simulink model "mult_signal"  (R2023a)
settings: Solver=FixedStepAuto  StartTime=0.0  StopTime=50.0  FixedStep=1e-5  RelTol=1e-3
undefined symbols (not defined in the file): LF, sample
libraries: instrumentseriallib x3
settings Model: Creator=Aliso  LastModifiedBy=Aliso

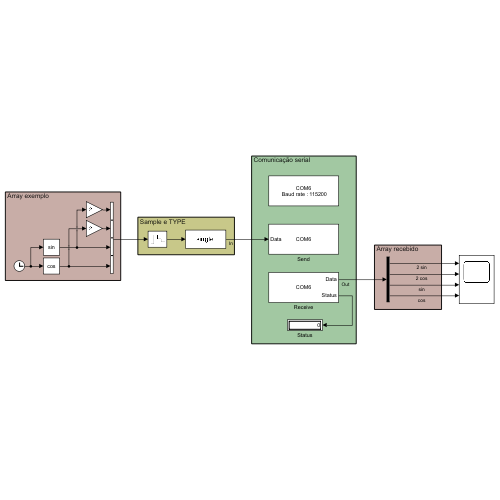
[thumbnail: Simulink's stored preview of the top-level diagram]
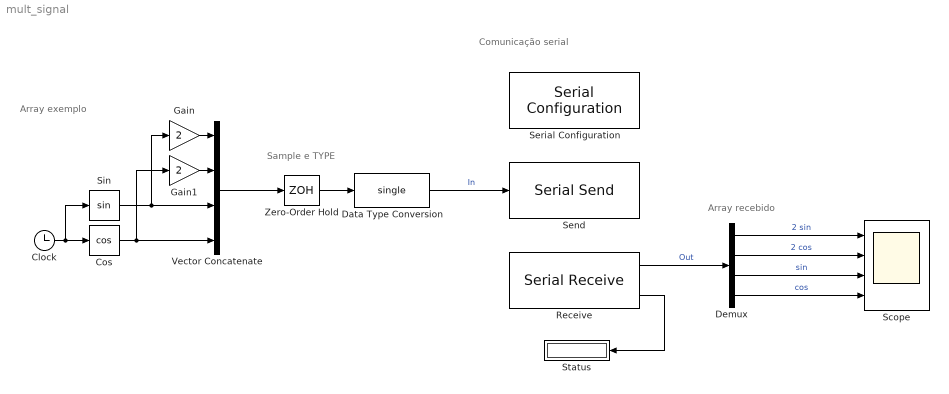
== system mult_signal ==
  note: Comunicação serial
  note: Array recebido
  note: Sample e TYPE
  note: Array exemplo
  Clock : Clock
  Cos : Trigonometry  Operator=cos
  Data Type Conversion : DataTypeConversion  OutDataTypeStr=single  SaturateOnIntegerOverflow=off  RndMeth=Floor  LockScale=on
  Demux : Demux
  Gain : Gain  Gain=2
  Gain1 : Gain  Gain=2
  Receive : instrumentseriallib/Serial Receive  Priority=1  PortSel=COM6  Port=COM6  ComPort=COM6  DataType=single  SaveDataType=uint8  ToggleHeader=on  Header=[65]  ToggleTerminator=on  Terminator=LF ('\n')  CustomTerminator=[]  InputFormat=Column major  ToggleDataSize=on  DataSize=[1 4]  EnableBlockingMode=off  ActionDataUnavailable=Output last received value  ActionWhenDataUnavailable=Output last received value  CustomValue=0  SampleTime=sample/2  SimulateUsing=Interpreted execution  BlockInModel=on  aMode=1
      settings: LibrarySourceBlock=c2000lib/Host Communication/Serial Receive
  Scope : Scope  NumInputPorts=4
  Send : instrumentseriallib/Serial Send  Priority=1  PortSel=COM6  Port=COM6  ComPort=COM6  Header=[65]  Terminator=LF ('\n')  CustomTerminator=[]  EnableBlockingMode=on  SimulateUsing=Interpreted execution  BlockInModel=on  aMode=1
      settings: LibrarySourceBlock=c2000lib/Host Communication/Serial Send
  Serial Configuration : instrumentseriallib/Serial Configuration  Priority=-200000  PortSel=COM6  Port=COM6  ComPort=COM6  BaudRate=115200  DataBits=8  Parity=none  StopBits=1  ByteOrder=little-endian  FlowControl=none  Timeout=10  SimulateUsing=Interpreted execution  BlockInModel=on  aMode=1
      settings: LibrarySourceBlock=c2000lib/Host Communication/Serial Configuration
  Sin : Trigonometry
  Status : Display
  Vector Concatenate : Concatenate  NumInputs=4
  Zero-Order Hold : ZeroOrderHold  SampleTime=sample
  wires:
  Vector Concatenate/1 -> Zero-Order Hold/1
  Zero-Order Hold/1 -> Data Type Conversion/1
  Receive/1 -> Demux/1  "Out"
  Demux/1 -> Scope/1  "2 sin"
  Demux/2 -> Scope/2  "2 cos"
  Demux/3 -> Scope/3  "sin"
  Demux/4 -> Scope/4  "cos"
  Receive/2 -> Status/1
  Data Type Conversion/1 -> Send/1  "In"
  Gain/1 -> Vector Concatenate/1
  Gain1/1 -> Vector Concatenate/2
  Sin/1 -> Gain/1, Vector Concatenate/3
  Cos/1 -> Gain1/1, Vector Concatenate/4
  Clock/1 -> Sin/1, Cos/1
